simulink model "avec_sat_op"  (R2024a)
settings: Solver=VariableStepAuto  StartTime=0.0  StopTime=800  RelTol=1e-3
settings Model: Creator=sabri  LastModifiedBy=sabri

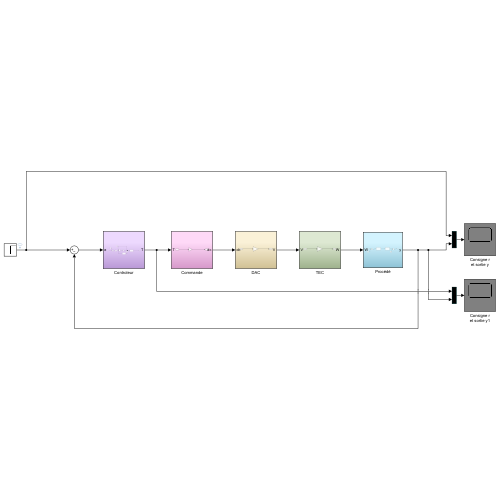
[thumbnail: Simulink's stored preview of the top-level diagram]
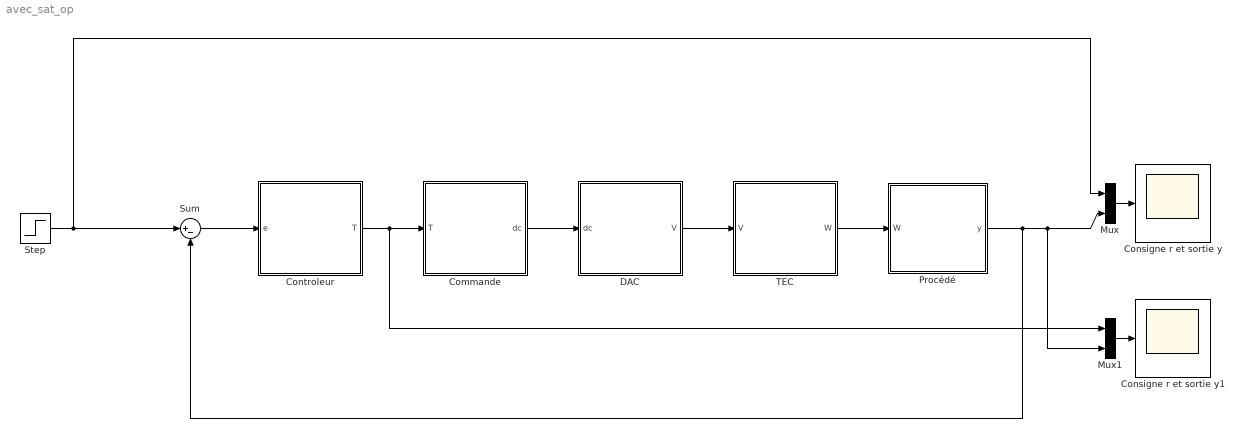
== system avec_sat_op ==
  Commande : Subsystem
  Consigne r et sortie y : Scope
  Consigne r et sortie y1 : Scope
  Controleur : Subsystem
  DAC : Subsystem
  Mux : Mux  Inputs=2
  Mux1 : Mux  Inputs=2
  Procédé : Subsystem
  Step : Step  Time=10  Before=23  After=33  SampleTime=0
  Sum : Sum  Inputs=|+-
  TEC : Subsystem
  wires:
  Mux/1 -> Consigne r et sortie y/1
  Sum/1 -> Controleur/1(e)
  Procédé/1(y) -> Sum/2, Mux1/2, Mux/2
  Step/1 -> Mux/1, Sum/1
  TEC/1(W) -> Procédé/1(W)
  Commande/1(dc) -> DAC/1(dc)
  DAC/1(V) -> TEC/1(V)
  Controleur/1(T) -> Mux1/1, Commande/1(T)
  Mux1/1 -> Consigne r et sortie y1/1

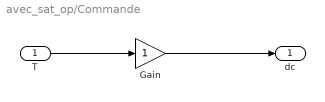
== system avec_sat_op/Commande ==
  T : Inport
  Gain : Gain
  dc : Outport
  wires:
  T/1 -> Gain/1
  Gain/1 -> dc/1

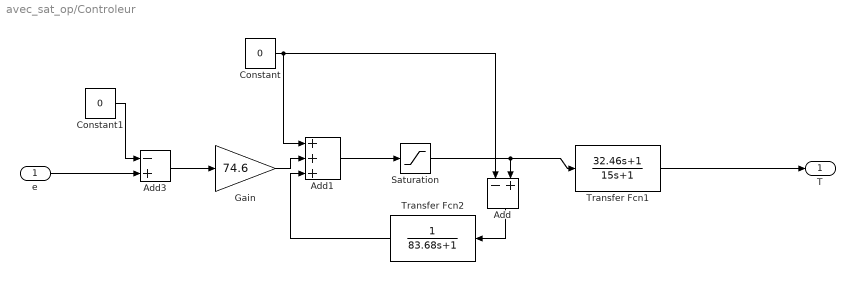
== system avec_sat_op/Controleur ==
  e : Inport
  Add : Sum  Inputs=-+
  Add1 : Sum  Inputs=+++
  Add3 : Sum  Inputs=-+
  Constant : Constant  Value=0
  Constant1 : Constant  Value=0
  Gain : Gain  Gain=74.6
  Saturation : Saturate  UpperLimit=100  LowerLimit=-100
  Transfer Fcn1 : TransferFcn  Numerator=[32.46 1]  Denominator=[15 1]
  Transfer Fcn2 : TransferFcn  Denominator=[83.68 1]
  T : Outport
  wires:
  e/1 -> Add3/2
  Constant1/1 -> Add3/1
  Transfer Fcn1/1 -> T/1
  Add3/1 -> Gain/1
  Gain/1 -> Add1/2
  Transfer Fcn2/1 -> Add1/3
  Add/1 -> Transfer Fcn2/1
  Constant/1 -> Add/1, Add1/1
  Add1/1 -> Saturation/1
  Saturation/1 -> Add/2, Transfer Fcn1/1

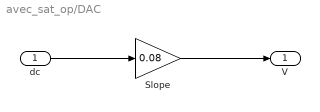
== system avec_sat_op/DAC ==
  dc : Inport
  Slope : Gain  Gain=0.08
  V : Outport
  wires:
  dc/1 -> Slope/1
  Slope/1 -> V/1

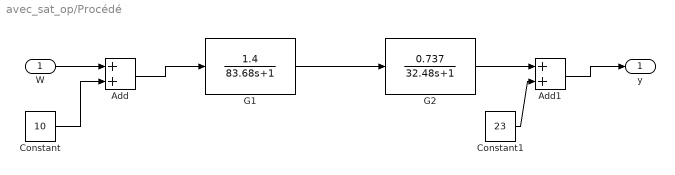
== system avec_sat_op/Procédé ==
  W : Inport
  Add : Sum
  Add1 : Sum
  Constant : Constant  Value=10
  Constant1 : Constant  Value=23
  G1 : TransferFcn  Numerator=[1.4]  Denominator=[83.68 1]
  G2 : TransferFcn  Numerator=[0.737]  Denominator=[32.48 1]
  y : Outport
  wires:
  G1/1 -> G2/1
  Add/1 -> G1/1
  W/1 -> Add/1
  Constant/1 -> Add/2
  G2/1 -> Add1/1
  Add1/1 -> y/1
  Constant1/1 -> Add1/2

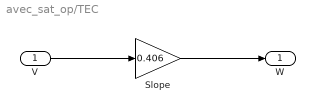
== system avec_sat_op/TEC ==
  V : Inport
  Slope : Gain  Gain=0.406
  W : Outport
  wires:
  Slope/1 -> W/1
  V/1 -> Slope/1
